simulink model "PD"  (R2020a)
settings: Solver=FixedStepAuto  StartTime=0.0  StopTime=89.99  FixedStep=0.001  RelTol=1e-3
undefined symbols (not defined in the file or in its folder): k_d, k_p
settings Model: Creator=lorenzoterenzi  LastModifiedBy=lorenzoterenzi

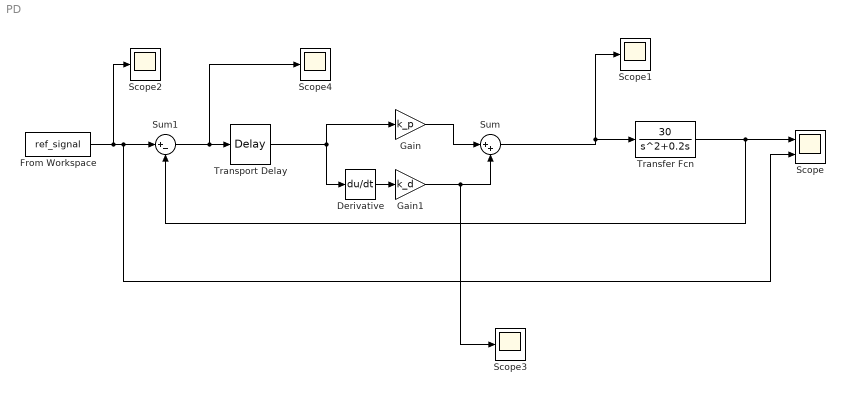
== system PD ==
  Derivative : Derivative
  From Workspace : FromWorkspace  VariableName=ref_signal
  Gain : Gain  Gain=k_p
  Gain1 : Gain  Gain=k_d
  Scope : Scope  NumInputPorts=2
  Scope{1..4} (4 alike) : Scope
  Sum : Sum  Inputs=|++
  Sum1 : Sum  Inputs=|+-
  Transfer Fcn : TransferFcn  Numerator=[30]  Denominator=[1 0.2 0]
  Transport Delay : TransportDelay  DelayTime=0.01  InitialOutput=0.00
  wires:
  From Workspace/1 -> Scope2/1, Scope/2, Sum1/1
  Derivative/1 -> Gain1/1
  Sum1/1 -> Scope4/1, Transport Delay/1
  Transport Delay/1 -> Derivative/1, Gain/1
  Gain/1 -> Sum/1
  Gain1/1 -> Scope3/1, Sum/2
  Transfer Fcn/1 -> Sum1/2, Scope/1
  Sum/1 -> Scope1/1, Transfer Fcn/1
